simulink model "a"  (R2023a)
settings: Solver=VariableStepAuto  StartTime=0.0  StopTime=10.0  RelTol=1e-3
settings Model: Creator=laura  LastModifiedBy=laura

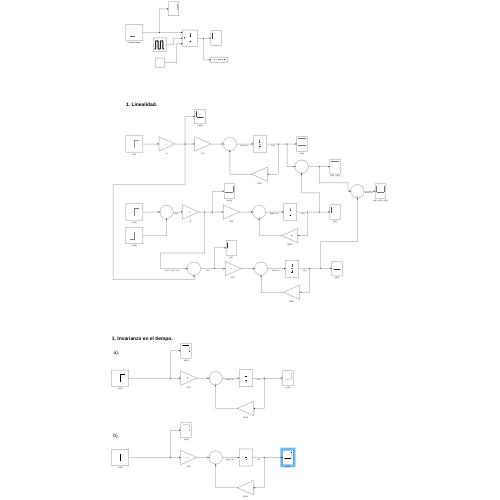
[thumbnail: Simulink's stored preview of the top-level diagram]
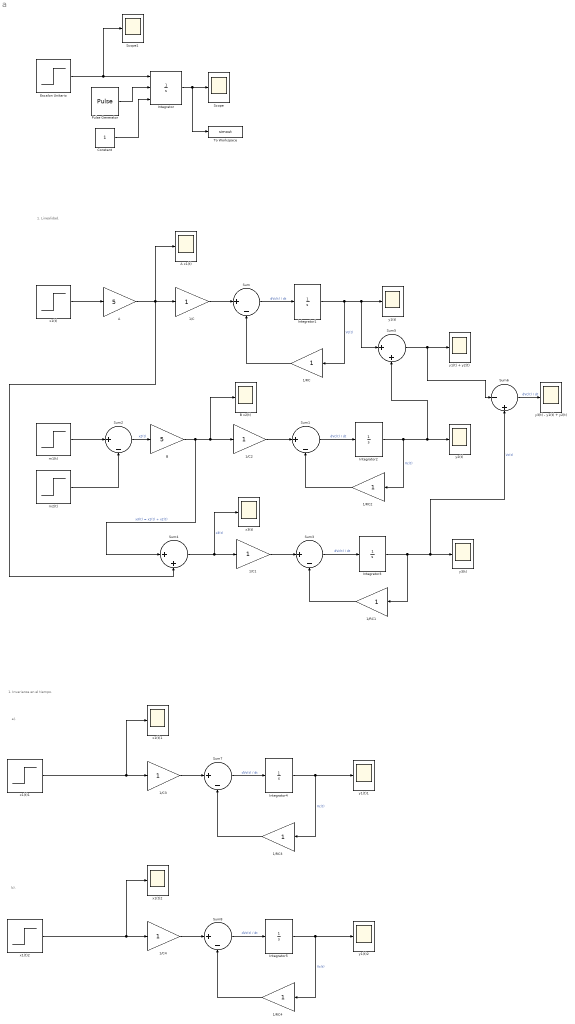
== system a ==
  note: a).
  note: 1. Linealidad.
  note: 1. Invarianza en el tiempo.
  note: b).
  " x1(t)1" : Scope
  " x1(t)2" : Scope
  1/C{,1..4} (5 alike) : Gain
  1/RC{,1..4} (5 alike) : Gain
  A : Gain  Gain=5
  A x1(t) : Scope
  B : Gain  Gain=5
  B x2(t) : Scope
  Constant : Constant
  Escalon Unitario : Step  SampleTime=0
  Integrator : Integrator  ExternalReset=rising  InitialConditionSource=external
  Integrator{1..5} (5 alike) : Integrator
  Pulse Generator : DiscretePulseGenerator  PulseType=Time based  Period=5  PulseWidth=50
  Scope : Scope
  Scope1 : Scope
  Sum{,1..3,7..8} (6 alike) : Sum  Inputs=|+-
  Sum4 : Sum  Inputs=|++
  Sum5 : Sum  Inputs=|++
  Sum6 : Sum  Inputs=|-+
  To Workspace : ToWorkspace  VariableName=simout  SaveFormat=Timeseries  SampleTime=-1
  m1(t) : Step  Time=0.8  After=0.9  SampleTime=0
  m2(t) : Step  SampleTime=0
  x1(t) : Step  SampleTime=0
  x1(t)1 : Step  SampleTime=0
  x1(t)2 : Step  Time=6  SampleTime=0
  x3(t) : Scope
  y1(t) : Scope
  y1(t) + y2(t) : Scope
  y1(t)1 : Scope
  y1(t)2 : Scope
  y2(t) : Scope
  y3(t) : Scope
  y3(t) - y1(t) + y2(t) : Scope
  wires:
  Escalon Unitario/1 -> Scope1/1, Integrator/1
  Integrator/1 -> To Workspace/1, Scope/1
  Pulse Generator/1 -> Integrator/2
  Constant/1 -> Integrator/3
  x1(t)/1 -> A/1
  A/1 -> 1/C/1, A x1(t)/1, Sum4/2
  1/C/1 -> Sum/1
  Sum/1 -> Integrator1/1  "dVc(t) / dt"
  Integrator1/1 -> 1/RC/1, Sum5/1, y1(t)/1  "Vc(t)"
  1/RC/1 -> Sum/2
  Sum1/1 -> Integrator2/1  "dVc(t) / dt"
  Integrator2/1 -> Sum5/2, y2(t)/1, 1/RC2/1  "Vc(t)"
  B/1 -> Sum4/1, 1/C2/1, B x2(t)/1  "x3(t) = x1(t) + x2(t)"
  1/C2/1 -> Sum1/1
  1/RC2/1 -> Sum1/2
  m1(t)/1 -> Sum2/1
  m2(t)/1 -> Sum2/2
  Sum2/1 -> B/1  "x2(t)"
  1/RC1/1 -> Sum3/2
  Sum3/1 -> Integrator3/1  "dVc(t) / dt"
  Integrator3/1 -> 1/RC1/1, Sum6/2, y3(t)/1  "Vc(t)"
  Sum4/1 -> 1/C1/1, x3(t)/1  "x3(t)"
  1/C1/1 -> Sum3/1
  Sum5/1 -> Sum6/1, y1(t) + y2(t)/1
  Sum6/1 -> y3(t) - y1(t) + y2(t)/1  "dVc(t) / dt"
  x1(t)1/1 -> 1/C3/1, " x1(t)1"/1
  Sum7/1 -> Integrator4/1  "dVc(t) / dt"
  1/RC3/1 -> Sum7/2
  1/C3/1 -> Sum7/1
  Integrator4/1 -> 1/RC3/1, y1(t)1/1  "Vc(t)"
  1/RC4/1 -> Sum8/2
  1/C4/1 -> Sum8/1
  Integrator5/1 -> 1/RC4/1, y1(t)2/1  "Vc(t)"
  x1(t)2/1 -> 1/C4/1, " x1(t)2"/1
  Sum8/1 -> Integrator5/1  "dVc(t) / dt"
